simulink model "rInvTemperatureDerate"  (R2024b)
settings: configuration reference "STM32H7_Config" (kept outside this file)
settings Model: DataDictionary=Master_Dictionary.sldd  EnableAccessToBaseWorkspace=off  Creator=torni  LastModifiedBy=William
settings ConfigSetRef: SourceName=STM32H7_Config

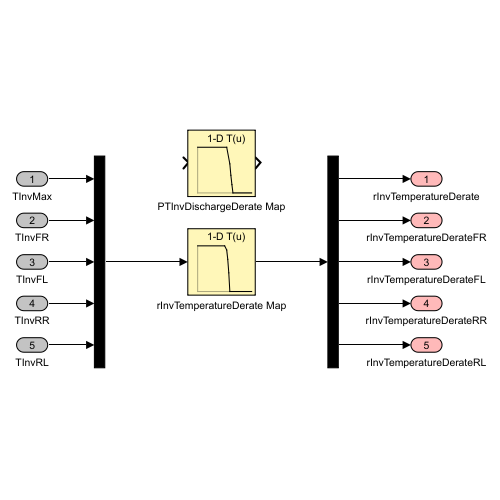
[thumbnail: Simulink's stored preview of the top-level diagram]
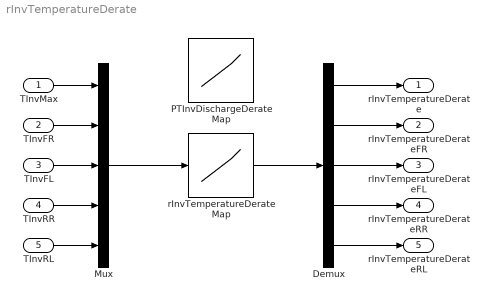
== system rInvTemperatureDerate ==
  "TInvMax " : Inport  OutDataTypeStr=double
  TInvFR : Inport  Port=2  OutDataTypeStr=double
  TInvFL : Inport  Port=3  OutDataTypeStr=double
  TInvRR : Inport  Port=4  OutDataTypeStr=double
  TInvRL : Inport  Port=5  OutDataTypeStr=double
  Demux : Demux  Outputs=5
  Mux : Mux  Inputs=5
  PTInvDischargeDerate Map : Lookup_n-D  NumberOfTableDimensions=1  BreakpointsForDimension1=[0,55,59,61,63,65,100]  Table=[80,80,50,30,15,0,0]  InternalRulePriority=Speed  RndMeth=Simplest
  rInvTemperatureDerate Map : Lookup_n-D  NumberOfTableDimensions=1  BreakpointsForDimension1=[0,50,54,56,58,60,100]  Table=[1,1,0.9,0.7,0.4,0,0]  InternalRulePriority=Speed  RndMeth=Simplest
  rInvTemperatureDerate : Outport  OutDataTypeStr=double  VectorParamsAs1DForOutWhenUnconnected=off
  rInvTemperatureDerateFR : Outport  Port=2  OutDataTypeStr=double  VectorParamsAs1DForOutWhenUnconnected=off
  rInvTemperatureDerateFL : Outport  Port=3  OutDataTypeStr=double  VectorParamsAs1DForOutWhenUnconnected=off
  rInvTemperatureDerateRR : Outport  Port=4  OutDataTypeStr=double  VectorParamsAs1DForOutWhenUnconnected=off
  rInvTemperatureDerateRL : Outport  Port=5  OutDataTypeStr=double  VectorParamsAs1DForOutWhenUnconnected=off
  wires:
  "TInvMax "/1 -> Mux/1
  TInvFR/1 -> Mux/2
  TInvFL/1 -> Mux/3
  TInvRR/1 -> Mux/4
  TInvRL/1 -> Mux/5
  Demux/5 -> rInvTemperatureDerateRL/1
  Demux/4 -> rInvTemperatureDerateRR/1
  Demux/3 -> rInvTemperatureDerateFL/1
  Demux/2 -> rInvTemperatureDerateFR/1
  Demux/1 -> rInvTemperatureDerate/1
  Mux/1 -> rInvTemperatureDerate Map/1
  rInvTemperatureDerate Map/1 -> Demux/1
